simulink model "Task2_TrafficLight"  (R2021a)
settings: Solver=FixedStepDiscrete  StartTime=0.0  StopTime=10.0  RelTol=1e-3  EnableMultiTasking=on
settings Model: SILPILModeSetting=veronly  ExtModeTrigDuration=2  Creator=Michael_Ibrahim  LastModifiedBy=Michael_Ibrahim
settings DataIOCC: ReturnWorkspaceOutputs=off
settings OptimizationCC: EnableMemcpy=off  LifeSpan=1  MaxStackSize=64  EfficientTunableParamExpr=on
settings DebuggingCC: UnderspecifiedInitializationDetection=Classic  MergeDetectMultiDrivingBlocksExec=none  SFMachineParentedDataDiag=warning  ArithmeticOperatorsInVariantConditions=warning
settings HardwareCC: ProdBitPerInt=16  ProdBitPerPointer=16  ProdBitPerSizeT=16  ProdBitPerPtrDiffT=16  ProdLargestAtomicFloat=None  ProdWordSize=8  ProdHWDeviceType=Atmel->AVR
settings ModelReferenceCC: PropagateSignalLabelsOutOfModel=off
settings SFSimCC: MATLABDynamicMemAlloc=off  CustomCodeUndefinedFunction=UseInterfaceOnly
settings RTWCC: SystemTargetFile=ert.tlc  HardwareBoard=Arduino Uno  GenCodeOnly=on  TemplateMakefile=ert_default_tmf  GenerateReport=on  Toolchain=Arduino AVR  IncludeHyperlinkInReport=on  LaunchReport=on  GenerateTraceInfo=on  GenerateTraceReport=on  GenerateTraceReportSl=on  GenerateTraceReportSf=on  GenerateTraceReportEml=on
settings CodeAppCC: ForceParamTrailComments=on  IgnoreCustomStorageClasses=off  OperatorAnnotations=on  SimulinkDataObjDesc=on  SFDataObjDesc=on  MATLABFcnDesc=on  InsertBlockDesc=on  StateflowObjectComments=on  MATLABSourceComments=on
settings ERTTargetCC: MultiwordLength=2048  SupportContinuousTime=on  SupportVariableSizeSignals=on  ExtModeStaticAllocSize=250

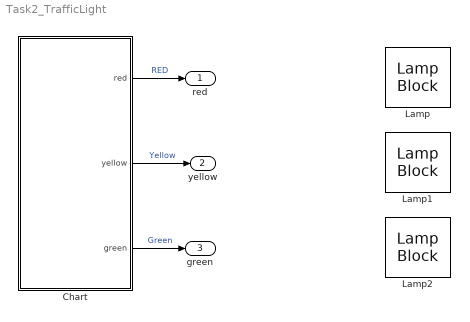
== system Task2_TrafficLight ==
  Chart : Stateflow chart  TreatAsAtomicUnit=on
  Lamp : LampBlock
  Lamp1 : LampBlock
  Lamp2 : LampBlock
  red : Outport
  yellow : Outport  Port=2
  green : Outport  Port=3
  wires:
  Chart/1(red) -> red/1  "RED"
  Chart/2(yellow) -> yellow/1  "Yellow"
  Chart/3(green) -> green/1  "Green"

== stateflow chart Task2_TrafficLight/Chart ==
  state RedLed
    en:
    red = uint8(0);
    yellow = uint8(0);
    green = uint8(0);
    du:
    red = uint8(1);
    yellow = uint8(0);
    green = uint8(0);
    ex:
    red = uint8(1);
    yellow = uint8(0);
    green = uint8(0);
  state YellowLed
    en:
    red = uint8(1);
    yellow = uint8(0);
    green = uint8(0);
    du:
    red = uint8(0);
    yellow = uint8(1);
    green = uint8(0);
    ex:
    red = uint8(0);
    yellow = uint8(1);
    green = uint8(0);
  state GreenLed
    en:
    red = uint8(0);
    yellow = uint8(1);
    green = uint8(0);
    du:
    red = uint8(0);
    yellow = uint8(0);
    green = uint8(1);
    ex:
    red = uint8(0);
    yellow = uint8(0);
    green = uint8(1);
  (default) -> RedLed
  RedLed -> YellowLed [order 1] : [after(3,sec)]
  YellowLed -> GreenLed : [after(3,sec)]
  RedLed -> GreenLed [order 2] : [after(3,sec)]
  data: data local; red output uint8; yellow output uint8; green output uint8
